simulink model "es4"  (R2022b)
settings: Solver=VariableStepAuto  StartTime=0.0  StopTime=10.0  RelTol=1e-3
undefined symbols (not defined in the file): A, B, C, D, denD, Derr, K, Nerr, numD, w
settings Model: Creator=emanuelevitetta  LastModifiedBy=emanuelevitetta

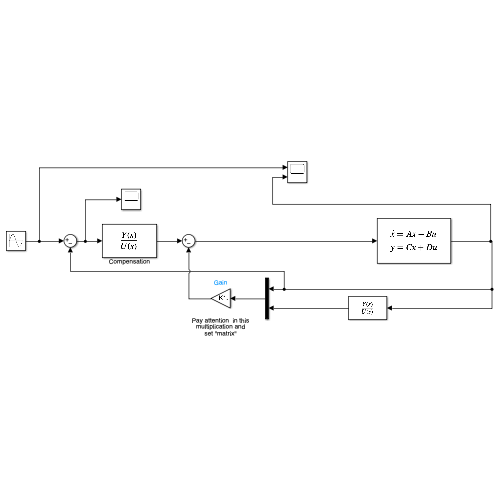
[thumbnail: Simulink's stored preview of the top-level diagram]
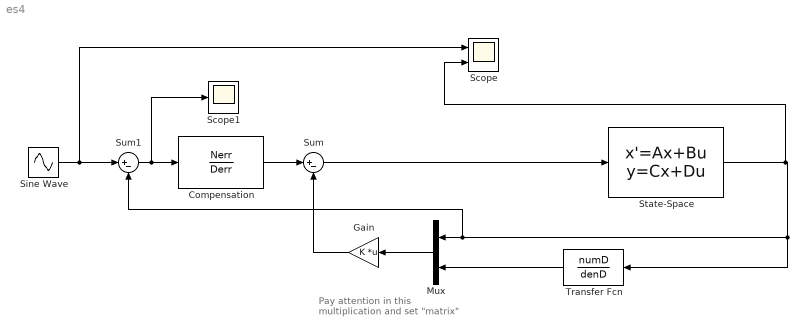
== system es4 ==
  note: Pay attention in this multiplication and set "matrix"
  Compensation : TransferFcn  Numerator=Nerr  Denominator=Derr
  Gain : Gain  Gain=K  Multiplication=Matrix(K*u)
  Mux : Mux  Inputs=2
  Scope : Scope  NumInputPorts=2
  Scope1 : Scope
  Sine Wave : Sin  Frequency=w  SampleTime=0
  State-Space : StateSpace  A=A  B=B  C=C  D=D  InitialCondition=0
  Sum : Sum  Inputs=|+-
  Sum1 : Sum  Inputs=|+-
  Transfer Fcn : TransferFcn  Numerator=numD  Denominator=denD
  wires:
  Compensation/1 -> Sum/1
  Mux/1 -> Gain/1
  Gain/1 -> Sum/2
  Sum/1 -> State-Space/1
  Sine Wave/1 -> Sum1/1, Scope/1
  State-Space/1 -> Scope/2, Transfer Fcn/1, Sum1/2, Mux/1
  Transfer Fcn/1 -> Mux/2
  Sum1/1 -> Scope1/1, Compensation/1
